simulink model "LPC"  (Simulink 5.0)
settings: Solver=FixedStepDiscrete  SolverMode=SingleTasking  StartTime=0.0  StopTime=inf  RelTol=1e-3
PreLoadFcn:
  | load mtlb;
libraries: dspstat3 x1, dspbuff3 x1, dspsigops x1, dspsolvers x1, dsparch4 x1, dspsrcs4 x1
settings Model: RequirementInfo=9  CovMetricSettings=d  Creator=dshpak  LastModifiedBy=Miky  ExtModeTrigMode=oneshot  ExtModeArmWhenConnect=off  ExtModeAutoUpdateStatusClock=off  SaveTime=off  SaveOutput=off  SaveFormat=Structure  LimitDataPoints=off  IntegerOverflowMsg=none  BlockReductionOpt=off  BooleanDataType=off  RTWOptions="-aEnforceIntegerDowncast=1 -aExtMode=0 -aExtModeTesting=0 -aFoldNonRolledExpr=1 -aForceParamTrailComments=0 -aGenerateComments=1 -aGenerateReport=0 -aIgnoreCustomStorageClasses=1 -aIncDataTypeInIds=0 -aIncHierarchyInIds=0 -aInlineInvariantSignals=0 -aInlinedPrmAccess=\"Literals\" -aLocalBlockOutputs=1 -aLogVarNameModifier=\"rt_\" -aMaxRTWIdLen=31 -aPrefixModelToSubsysFcnNames=1 -aRTWVerbose=1 -aRollThreshold=5 -aShowEliminatedStatements=1"

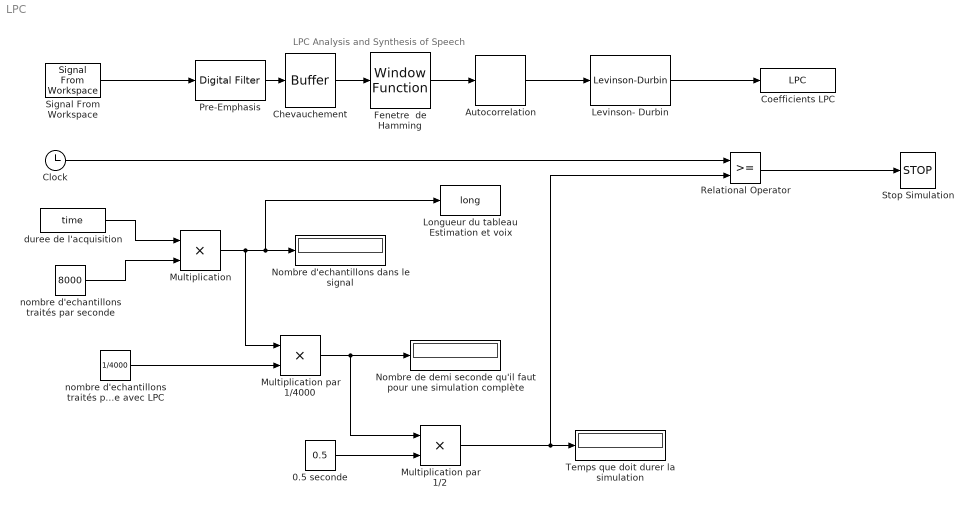
== system LPC ==
  note: LPC Analysis and Synthesis of Speech
  0.5 seconde : Constant  Value=0.5
  Autocorrelation : dspstat3/Autocorrelation  AllPositiveLags=off  maxlag=12  bias=Biased  domain=Time
  Chevauchement : dspbuff3/Buffer  N=160  V=80  ic=0
  Clock : Clock
      settings: Decimation=10
  Coefficients LPC : ToWorkspace  VariableName=LPC  SampleTime=-1  SaveFormat=Array
  Fenetre  de Hamming : dspsigops/Window Function  winmode=Apply window to input  wintype=Hamming  N=64  Rs=50  beta=10  winsamp=Symmetric  UserWindow=hamming  OptParams=off  UserParams={1.0}  datatype=Double
  Levinson- Durbin : dspsolvers/Levinson-Durbin  coeffOutFcn=A  outP=off  zeroInpHandling=on
  Longueur du tableau Estimation et voix : ToWorkspace  VariableName=long  SampleTime=-1  SaveFormat=StructureWithTime
      settings: MaxDataPoints=1
  Multiplication : Product  Inputs=**  ShowAdditionalParam=on  OutDataTypeMode=single  OutScaling=2^-10
  Multiplication par 1/2 : Product  Inputs=**  ShowAdditionalParam=on  OutDataTypeMode=double  OutScaling=2^-10
  Multiplication par 1/4000 : Product  Inputs=**  OutDataTypeMode=single  OutScaling=2^-10
  Nombre d'echantillons dans le signal : Display
  Nombre de demi seconde qu'il faut pour une simulation complète : Display
  Pre-Emphasis : dsparch4/Digital Filter  TypePopup=FIR (all zeros)  IIRFiltStruct=Direct form II transposed  AllPoleFiltStruct=Direct form  FIRFiltStruct=Direct form  CoeffSource=Specify via dialog  NumCoeffs=[1 -.95]  DenCoeffs=[1 0.1]  BiQuadCoeffs=[1 0.3 0.4 1 0.1 0.2]  LatticeCoeffs=[0.2 0.4]  denIgnore=on  FiltPerSampPopup=One filter per frame  IC=0  ICnum=0  ICden=0
  Relational Operator : RelationalOperator
  Signal From Workspace : dspsrcs4/Signal From Workspace  X=voix  Ts=1/8000  nsamps=160  OutputAfterFinalValue=Setting to zero
  Stop Simulation : Stop
  Temps que doit durer la simulation : Display
  duree de l'acquisition : FromWorkspace  VariableName=time  SampleTime=0
  nombre d'echantillons traités par 0.5 seconde avec LPC : Constant  Value=1/4000
  nombre d'echantillons traités par seconde : Constant  Value=8000  ShowAdditionalParam=on  OutDataTypeMode=double
  wires:
  Autocorrelation/1 -> Levinson- Durbin/1
  Fenetre  de Hamming/1 -> Autocorrelation/1
  Levinson- Durbin/1 -> Coefficients LPC/1
  Signal From Workspace/1 -> Pre-Emphasis/1
  Pre-Emphasis/1 -> Chevauchement/1
  Chevauchement/1 -> Fenetre  de Hamming/1
  Clock/1 -> Relational Operator/1
  Relational Operator/1 -> Stop Simulation/1
  nombre d'echantillons traités par seconde/1 -> Multiplication/2
  Multiplication/1 -> Multiplication par 1/4000/1, Nombre d'echantillons dans le signal/1, Longueur du tableau Estimation et voix/1
  Multiplication par 1/4000/1 -> Nombre de demi seconde qu'il faut pour une simulation complète/1, Multiplication par 1/2/1
  nombre d'echantillons traités par 0.5 seconde avec LPC/1 -> Multiplication par 1/4000/2
  0.5 seconde/1 -> Multiplication par 1/2/2
  Multiplication par 1/2/1 -> Temps que doit durer la simulation/1, Relational Operator/2
  duree de l'acquisition/1 -> Multiplication/1
